simulink model "verify_EU_Tapping_mdl"  (Simulink 8.2)
settings: Solver=ode45  StartTime=0.0  StopTime=24*3600  MaxStep=60  RelTol=1e-3
libraries: carnot x6
settings Model: Creator=drhf  LastModifiedBy=drhf
settings DataIOCC: MaxDataPoints=1

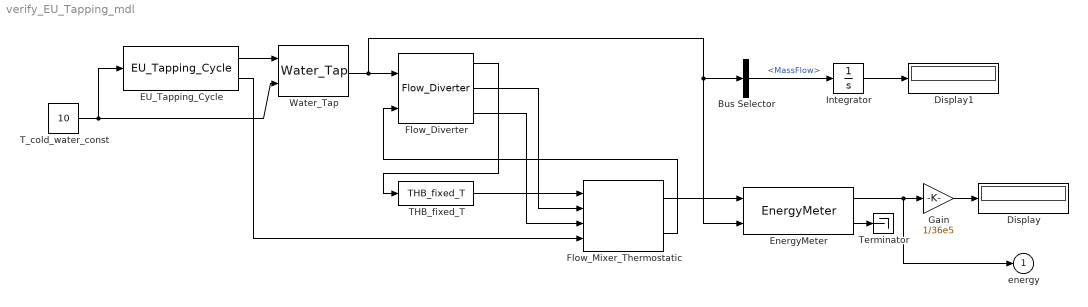
== system verify_EU_Tapping_mdl ==
  Bus Selector : BusSelector  OutputSignals=MassFlow
  Display : Display
  Display1 : Display
  EU_Tapping_Cycle : carnot/Load/Hot_Water_Tapping/EU_Tapping_Cycle  eu_tap=4XL
  EnergyMeter : carnot/Control/EnergyMeter
  Flow_Diverter : carnot/Hydraulics/Flow_Diverter
  Flow_Mixer_Thermostatic : carnot/Hydraulics/Flow_Mixer_Thermostatic  t=10
  Gain : Gain  Gain=1/36e5
  Integrator : Integrator
  THB_fixed_T : carnot/Source/Simple/THB_fixed_T  t=60
  T_cold_water_const : Constant  Value=10
  Terminator : Terminator
  Water_Tap : carnot/Load/Hot_Water_Tapping/Water_Tap  dia=0.02  p=2e5
  energy : Outport  InitialOutput=0
  wires:
  EnergyMeter/1 -> Gain/1, energy/1
  Gain/1 -> Display/1
  Water_Tap/1 -> Bus Selector/1, EnergyMeter/2, Flow_Diverter/1
  T_cold_water_const/1 -> EU_Tapping_Cycle/1, Water_Tap/2
  EU_Tapping_Cycle/1 -> Water_Tap/1
  EU_Tapping_Cycle/2 -> Flow_Mixer_Thermostatic/4
  Flow_Diverter/3 -> Flow_Mixer_Thermostatic/3
  Flow_Diverter/2 -> Flow_Mixer_Thermostatic/2
  THB_fixed_T/1 -> Flow_Mixer_Thermostatic/1
  Flow_Mixer_Thermostatic/1 -> EnergyMeter/1
  Flow_Mixer_Thermostatic/2 -> Flow_Diverter/2
  Flow_Diverter/1 -> THB_fixed_T/1
  Bus Selector/1 -> Integrator/1  "<MassFlow>"
  Integrator/1 -> Display1/1
  EnergyMeter/2 -> Terminator/1
